simulink model "filter0"  (R2020b)
settings: Solver=VariableStepAuto  StartTime=0.0  StopTime=10.0  RelTol=1e-3
settings Model: Creator=Lenovo  LastModifiedBy=Lenovo
settings DataIOCC: SaveOutput=off  SaveTime=off

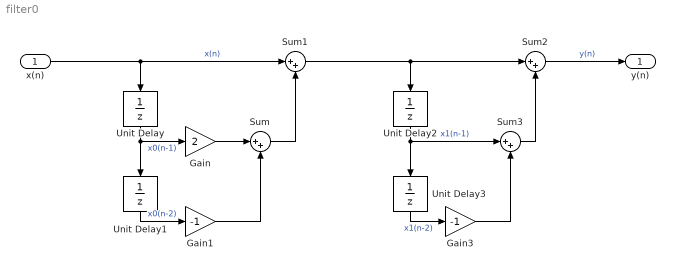
== system filter0 ==
  x(n) : Inport  OutDataTypeStr=double  PortDimensions=1  SampleTime=0
  Gain : Gain  Gain=2
  Gain1 : Gain  Gain=-1
  Gain3 : Gain  Gain=-1
  Sum{,1..3} (4 alike) : Sum  Inputs=|++
  Unit Delay{,1..3} (4 alike) : UnitDelay  SampleTime=-1  HasFrameUpgradeWarning=on
  y(n) : Outport  OutDataTypeStr=double  PortDimensions=1  SampleTime=0
  wires:
  Gain1/1 -> Sum/2
  Unit Delay1/1 -> Gain1/1  "x0(n-2)"
  Unit Delay2/1 -> Sum3/1, Unit Delay3/1  "x1(n-1)"
  x(n)/1 -> Sum1/1, Unit Delay/1  "x(n)"
  Unit Delay3/1 -> Gain3/1  "x1(n-2)"
  Gain3/1 -> Sum3/2
  Sum/1 -> Sum1/2
  Sum2/1 -> y(n)/1  "y(n)"
  Gain/1 -> Sum/1
  Unit Delay/1 -> Unit Delay1/1, Gain/1  "x0(n-1)"
  Sum1/1 -> Unit Delay2/1, Sum2/1
  Sum3/1 -> Sum2/2
